simulink model "es2_ACPC_sim"  (R2022b)
settings: Solver=VariableStepAuto  StartTime=0.0  StopTime=10000  RelTol=1e-3
values from neighbouring files (symbols this model uses):
  alfa = 7.29    [ES2.m]
  beta = 1    [ES2.m]
  delta = 10    [ES2.m]
  K = 10    [ES2.m]
settings Model: Creator=claudio  LastModifiedBy=claudio

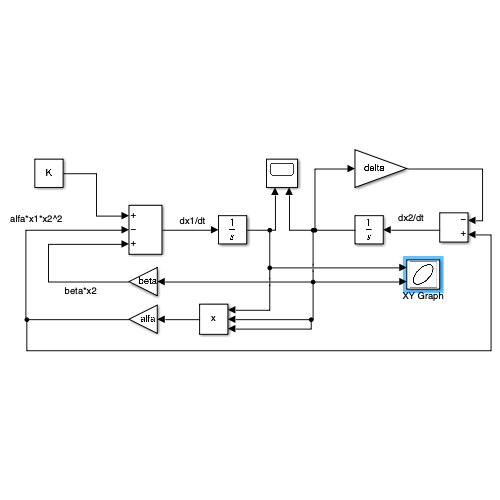
[thumbnail: Simulink's stored preview of the top-level diagram]
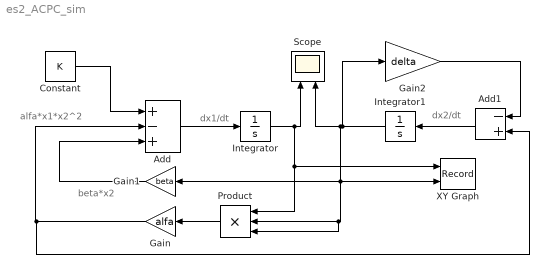
== system es2_ACPC_sim ==
  note: dx2/dt
  note: beta*x2
  note: dx1/dt
  note: alfa*x1*x2^2
  Add : Sum  Inputs=+-+
  Add1 : Sum  Inputs=-+
  Constant : Constant  Value=K
  Gain : Gain  Gain=alfa
  Gain1 : Gain  Gain=beta
  Gain2 : Gain  Gain=delta
  Integrator : Integrator
  Integrator1 : Integrator
  Product : Product  Inputs=3
  Scope : Scope  NumInputPorts=2
  XY Graph : Record  FileSettingsInternal="{\"entries\":[{\"content\":{\"excelSettings\":{\"content\":{},\"type\":\"Streamout.ExcelSettings\"}},\"type\":\"Streamout.FileSettingStorage\",\"uuid\":\"e70cfc5e-6016-4b95-9ca2-9922e4996af1\"}],\"packageUris\":[\"http://schema.mathworks.com/mf0/streamout_blocks/R2020a\"],\"version\":\"1.0\"}"  Layout=[1 1]  SignalsInternal="{\"entries\":[{\"content\":{\"signals\":[{\"content\":{\"blockPath\":[\"es2_ACPC_sim/XY Graph\"],\"channel\":[],\"dimensions\":[1],\"domain\":\"es2_ACPC_sim/XY Graph\",\"lineColor\":\"#a2142f\",\"plots\":[1],\"port\":1,\"sid\":[\"\"],\"signalID\":89,\"signalName\":\"Integrator\"},\"type\":\"RecordBlkView.Signal\",\"uuid\":\"b0f3f79c-7d41-4bea-85f7-72b89eacba0c\"},{\"content\":{\"blockPath\":[\"es2_ACPC_sim/XY Graph\"],\"channel\":[],\"dimensions\":[1],\"domain\":\"es2_ACPC_sim/XY Graph\",\"lineColor\":\"#139fff\",\"plots\":[1],\"port\":2,\"sid\":[\"\"],\"signalID\":93,\"signalName\":\"Integrator1\"},\"type\":\"RecordBlkView.Signal\",\"uuid\":\"1e7a468e-7206-4b83-9d00-9f80901c460e\"}]},\"type\":\"RecordBlkView.InputSignals\",\"uuid\":\"5d3ba0ae-a410-4d66-a412-0e8d730796e1\"}],\"packageUris\":[\"http://schema.mathworks.com/mf0/streamout_blocks/R2020a\"],\"version\":\"1.0\"}"  VisualizationBindings="{\"xyplotplugin\":{\"info\":[{\"series\":[{\"bindingParametersList\":[{\"parameter\":\"X-Axis\",\"signalID\":89,\"signalName\":\"Integrator\"},{\"parameter\":\"Y-Axis\",\"signalID\":93,\"signalName\":\"Integrator1\"}],\"seriesID\":35740}],\"subplotID\":1}]}}"  CompatibilityTag=XY
  wires:
  Add/1 -> Integrator/1
  Constant/1 -> Add/1
  Gain/1 -> Add1/2, Add/2
  Product/1 -> Gain/1
  Integrator/1 -> Product/1, XY Graph/1, Scope/1
  Gain1/1 -> Add/3
  Add1/1 -> Integrator1/1
  Integrator1/1 -> Scope/2, Product/3, Product/2, XY Graph/2, Gain1/1, Gain2/1
  Gain2/1 -> Add1/1
